simulink model "rmsdemo"  (Simulink 2.20)
settings: Solver=ode45  SolverMode=SingleTasking  StartTime=0.0  StopTime=10.0  RelTol=1e-8  AbsTol=1e-10
settings Model: SaveTime=off  SaveOutput=off  ConsistencyChecking=off  RTWPlaceOutputsASAP=off  RTWLocalBlockOutputs=on  ExtModeTrigMode=oneshot

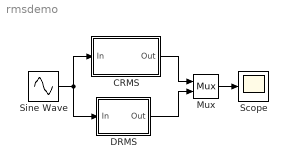
== system rmsdemo ==
  CRMS : Subsystem
      mask Type: Continuous RMS Value Block
      mask Description: Computes the cumulative root mean squared value of the input signal. The output is continuous.
      mask Display: disp('Continuous\nRMS');
  DRMS : Subsystem  mask(Discrete RMS Value Block){Ts=0.5}
      mask prompts: Ts "Sampling Interval (s) :"
      mask help: Computes the cumulative root mean squared value of the sampled input input signal. The output is discrete.
      mask Display: disp('Discrete\nRMS')
  Mux : Mux  Inputs=2
      settings: DisplayOption=none
  Scope : Scope
      settings: TickLabels=on  Titles=%s  TimeRange=auto  YMin=0  YMax=1  SaveToWorkspace=off  SaveName=ScopeData  DataFormat=matrix
  Sine Wave : Sin  Amplitude=1  Frequency=1  Phase=0  SampleTime=0
  wires:
  Sine Wave/1 -> CRMS/1(In), DRMS/1(In)
  DRMS/1(Out) -> Mux/2
  CRMS/1(Out) -> Mux/1
  Mux/1 -> Scope/1

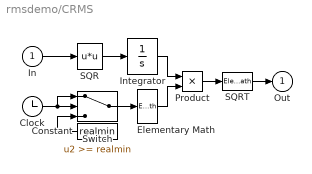
== system rmsdemo/CRMS ==
  In : Inport  Port=1  PortWidth=-1  SampleTime=-1
  Clock : Clock
      settings: DisplayTime=off  Decimation=10
  Constant : Constant  Orientation=left  Value=realmin
  Elementary Math : ElementaryMath  Operator=reciprocal
  Integrator : Integrator  ExternalReset=none  InitialConditionSource=internal  InitialCondition=0  LimitOutput=on  UpperSaturationLimit=inf  LowerSaturationLimit=0  ShowSaturationPort=off  ShowStatePort=off  AbsoluteTolerance=auto
  Product : Product  Inputs=2
  SQR : Fcn  Expr=u*u
  SQRT : ElementaryMath  Operator=sqrt
  Switch : Switch  Threshold=realmin
  Out : Outport  Port=1  InitialOutput=0
  wires:
  In/1 -> SQR/1
  SQR/1 -> Integrator/1
  Integrator/1 -> Product/1
  Switch/1 -> Elementary Math/1
  Clock/1 -> Switch/2, Switch/1
  Constant/1 -> Switch/3
  Elementary Math/1 -> Product/2
  SQRT/1 -> Out/1
  Product/1 -> SQRT/1

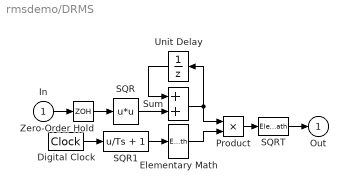
== system rmsdemo/DRMS ==
  In : Inport  Port=1  PortWidth=-1  SampleTime=-1
  Digital Clock : DigitalClock  SampleTime=Ts
  Elementary Math : ElementaryMath  Operator=reciprocal
  Product : Product  Inputs=2
  SQR : Fcn  Expr=u*u
  SQR1 : Fcn  Expr=u/Ts + 1
  SQRT : ElementaryMath  Operator=sqrt
  Sum : Sum  Inputs=++
  Unit Delay : UnitDelay  Orientation=left  X0=0  SampleTime=Ts
  Zero-Order Hold : ZeroOrderHold  SampleTime=Ts
  Out : Outport  Port=1  InitialOutput=0
  wires:
  SQR1/1 -> Elementary Math/1
  Digital Clock/1 -> SQR1/1
  SQRT/1 -> Out/1
  Product/1 -> SQRT/1
  Elementary Math/1 -> Product/2
  Unit Delay/1 -> Sum/1
  Sum/1 -> Unit Delay/1, Product/1
  SQR/1 -> Sum/2
  Zero-Order Hold/1 -> SQR/1
  In/1 -> Zero-Order Hold/1
